simulink model "oldVers_1704_old"  (R2023a)
settings: Solver=ode1  StartTime=0.0  StopTime=0.5  FixedStep=0.000001  RelTol=1e-3
values from neighbouring files (symbols this model uses):
  Cm = 0.05    [matlab2.mat]
  Jm = 1    [matlab2.mat]
  k_eq = 1    [matlab2.mat]
  k_pos = 1    [matlab2.mat]
  Ki_Curr = 1666    [matlab2.mat]
  Kinv = 18    [matlab2.mat]
  Kp_Curr = 0.0229017    [matlab2.mat]
  Re = 0.357267    [matlab2.mat]
  T_eq = 0.00052    [matlab2.mat]
  T_eq2 = 0.0018    [matlab2.mat]
  Te = 0.0006    [matlab2.mat]
  Tinv = 0.00026    [matlab2.mat]
undefined symbols (not defined in the file or in its folder): Kc_Curr, Kc_Pos, Kc_Speed, Kis_Curr
libraries: simulink x3
settings Model: Creator=Ruslan  LastModifiedBy=sokur
settings SolverCC: AlgebraicLoopSolver=TrustRegion
settings ModelReferenceCC: EnableRefExpFcnMdlSchedulingChecks=on

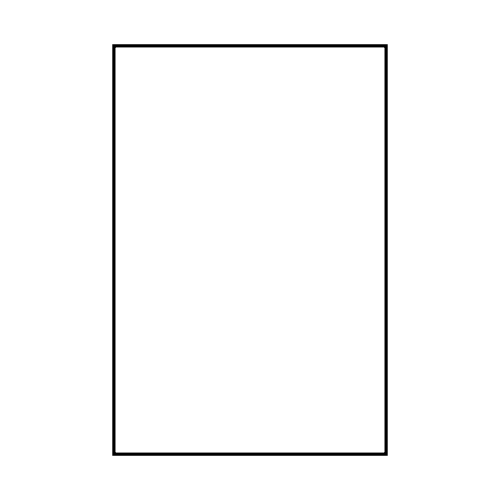
[thumbnail: Simulink's stored preview of the top-level diagram]
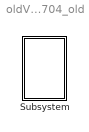
== system oldVers_1704_old ==
  Subsystem : Subsystem

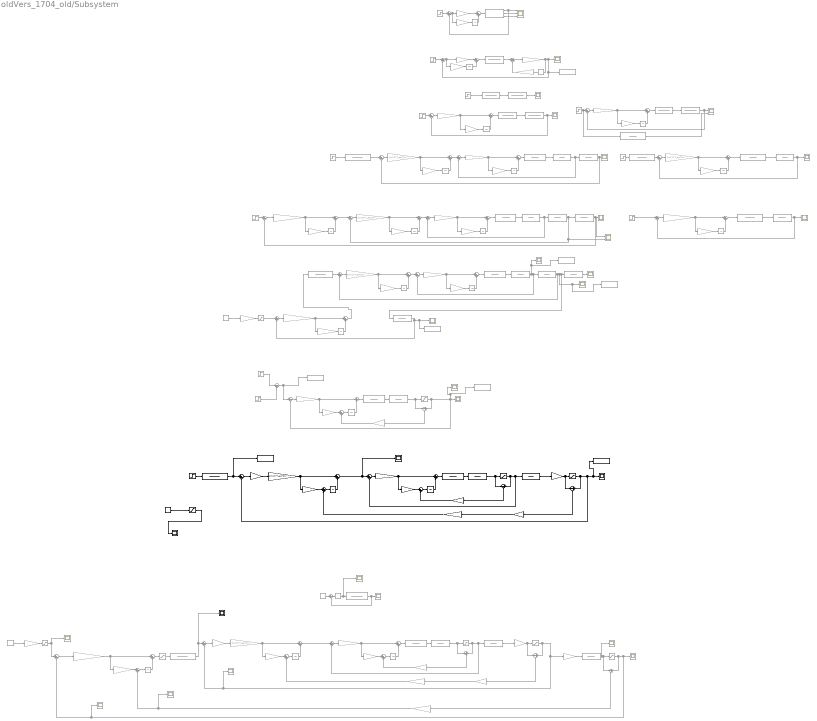
== system oldVers_1704_old/Subsystem ==
  note: Контур скорости с насыщениями рабочий
  note: Контур тока с ограничениями рабочий
  note: Контур положения рабочий
  note: Контур скорости
  note: Контур тока
  note: Контур тока
  note: Контур тока рабочий
  1 : TransferFcn  Commented=on  Numerator=[Cm]  Denominator=[Jm 0]
  1/Rяц : Gain  Commented=on  Gain=1/0.357267
  2 : TransferFcn  Commented=on  Numerator=[k_pos]  Denominator=[1 0]
  3 : TransferFcn  Commented=on  Numerator=[k_pos]  Denominator=[1 0]
  Constant : Constant  Commented=on  Value=20
  Derivative : Derivative  Commented=on
  Integrator{,1..14,19..20,22} (18 alike) : Integrator  Commented=on
  Integrator16 : Integrator
  Integrator18 : Integrator
  Kп : Gain  Commented=on  Gain=0.00067
  Kп1 : Gain  Commented=on  Gain=0.00067
  Kп{6,10..11,32} (4 alike) : Gain  Commented=on  Gain=(1)/(2*T_eq2*k_pos)
  Kп{3,8,12..13,25} (5 alike) : Gain  Commented=on  Gain=Kp_Curr
  Kп{4,7,9,14,27} (5 alike) : Gain  Commented=on  Gain=(Jm)/(2*T_eq*Cm)
  Kп2 : Gain  Commented=on  Gain=0.0229017
  Kп20 : Gain  Gain=Kp_Curr
  Kп21 : Gain  Gain=30/pi
  Kп22 : Gain  Gain=(Jm)/(2*T_eq*Cm)
  Kп23 : Gain  Gain=1/(30/pi)
  Kп24 : Gain  Gain=1/(30/pi)
  Kп26 : Gain  Commented=on  Gain=30/pi
  Kп28 : Gain  Commented=on  Gain=1/(30/pi)
  Kп29 : Gain  Commented=on  Gain=1/(30/pi)
  Kп33 : Gain  Commented=on  Gain=1/(30/pi)
  Kп5 : Gain  Commented=on  Gain=0.0229017
  L : Gain  Commented=on  Gain=0.001457602
  Ramp1 : simulink/Sources/Ramp  Commented=on  slope=120  start=0  InitialOutput=0
  Ramp2 : simulink/Sources/Ramp  Commented=on  slope=10000  start=0  InitialOutput=0
  Ramp3 : simulink/Sources/Ramp  slope=7500  start=0  InitialOutput=0
  Relay : Relay  Commented=on  OnOutputValue=20  OffOutputValue=-20
  Saturation : Saturate  Commented=on  UpperLimit=70  LowerLimit=-70
  Saturation1 : Saturate  Commented=on  UpperLimit=48  LowerLimit=-48
  Saturation10 : Saturate  UpperLimit=750  LowerLimit=-750
  Saturation2 : Saturate  Commented=on  UpperLimit=2000  LowerLimit=-2000
  Saturation4 : Saturate  UpperLimit=70  LowerLimit=-70
  Saturation5 : Saturate  UpperLimit=750  LowerLimit=-750
  Saturation6 : Saturate  Commented=on  UpperLimit=70  LowerLimit=-70
  Saturation7 : Saturate  Commented=on  UpperLimit=750  LowerLimit=-750
  Saturation8 : Saturate  Commented=on  UpperLimit=96  LowerLimit=-40
  Saturation9 : Saturate  Commented=on  UpperLimit=90  LowerLimit=-90
  Scope : Scope  Commented=on  NumInputPorts=3
  Scope{1..4,6..9,11..13,15..19,21,23..26} (21 alike) : Scope  Commented=on
  Scope10 : Scope  Commented=on  NumInputPorts=2
  Scope{14,20,22,27} (4 alike) : Scope
  Scope5 : Scope  Commented=on  NumInputPorts=2
  Step : Step  Commented=on  Time=0  After=-12  SampleTime=0
  Step{1..7,9} (8 alike) : Step  Commented=on  Time=0  SampleTime=0
  Step10 : Step  Commented=on  Time=0.0017  After=50  SampleTime=0
  Step11 : Step  Time=0  After=700  SampleTime=0
  Step8 : Step  Commented=on  Time=0  After=100  SampleTime=0
  Sum{,2,6,8..9,12,15..16,19..20,22,24,27..28,30,34,51,55,63} (19 alike) : Sum  Commented=on  Inputs=|+-
  Sum{1,3,5,7,10..11,13..14,17..18,21,23,25..26,29,31,50,52,54,56,62,65} (22 alike) : Sum  Commented=on  Inputs=|++
  Sum{32,53,57,64} (4 alike) : Sum  Commented=on  Inputs=-|+
  Sum33 : Sum  Commented=on  Inputs=|-+
  Sum4 : Sum  Commented=on  Inputs=-+-
  Sum{42,44,46,48} (4 alike) : Sum  Inputs=|++
  Sum43 : Sum  Inputs=|+-
  Sum45 : Sum  Inputs=-|+
  Sum47 : Sum  Inputs=|+-
  Sum49 : Sum  Inputs=-|+
  To Workspace : ToWorkspace  Commented=on  VariableName=simout  SaveFormat=Timeseries  SampleTime=-1
  To Workspace1 : ToWorkspace  Commented=on  VariableName=pos  SaveFormat=Timeseries  SampleTime=-1
  To Workspace2 : ToWorkspace  Commented=on  VariableName=posCurr  SaveFormat=Timeseries  SampleTime=-1
  To Workspace3 : ToWorkspace  Commented=on  VariableName=posSpd  SaveFormat=Timeseries  SampleTime=-1
  To Workspace4 : ToWorkspace  Commented=on  VariableName=CurrC  SaveFormat=Timeseries  SampleTime=-1
  To Workspace5 : ToWorkspace  Commented=on  VariableName=CurrCRef  SaveFormat=Timeseries  SampleTime=-1
  To Workspace6 : ToWorkspace  VariableName=SpdC  SaveFormat=Timeseries  SampleTime=-1
  To Workspace7 : ToWorkspace  VariableName=SpdCRef  SaveFormat=Timeseries  SampleTime=-1
  Transfer Fcn : TransferFcn  Commented=on  Denominator=[Kis_Curr 0]
  Аппроксимация ЗКС : TransferFcn  Commented=on  Denominator=[T_eq2 1]
  Аппроксимация ЗКТ : TransferFcn  Commented=on  Numerator=[k_eq]  Denominator=[T_eq 1]
  Аппроксимация ЗКТ1 : TransferFcn  Commented=on  Denominator=[T_eq 1]
  Аппроксимация ЗКТ3 : TransferFcn  Commented=on  Denominator=[4*T_eq 1]
  ДПТ : Subsystem  Commented=on
  Инвентор : TransferFcn  Commented=on  Numerator=[617.143]  Denominator=[0.00026 1]
  Инвентор1 : TransferFcn  Commented=on  Numerator=[18]  Denominator=[0.00026 1]
  Инвентор{3,5..6,8,10} (5 alike) : TransferFcn  Commented=on  Numerator=[Kinv]  Denominator=[Tinv 1]
  Инвентор2 : TransferFcn  Commented=on  Numerator=[18]  Denominator=[0.00026 1]
  Инвентор4 : TransferFcn  Commented=on  Numerator=[18]  Denominator=[0.00026 1]
  Инвентор9 : TransferFcn  Numerator=[Kinv]  Denominator=[Tinv 1]
  Ки : Gain  Commented=on  Gain=0.22167
  Ки1 : Gain  Commented=on  Gain=0.22167
  Ки{6,10..11,31} (4 alike) : Gain  Commented=on  Gain=1/(4*T_eq2)
  Ки12 : Gain  Commented=on  Gain=Kc_Curr
  Ки{3,8,13..14,26} (5 alike) : Gain  Commented=on  Gain=Ki_Curr
  Ки{4,7,9,15,28} (5 alike) : Gain  Commented=on  Gain=1/(4*T_eq)
  Ки16 : Gain  Commented=on  Gain=1/k_pos
  Ки2 : Gain  Commented=on  Gain=1666
  Ки21 : Gain  Gain=Kc_Curr
  Ки22 : Gain  Gain=Ki_Curr
  Ки23 : Gain  Gain=Kc_Speed
  Ки24 : Gain  Gain=1/(4*T_eq)
  Ки25 : Gain  Commented=on  Gain=Kc_Curr
  Ки27 : Gain  Commented=on  Gain=Kc_Speed
  Ки29 : Gain  Commented=on  Gain=1/k_pos
  Ки32 : Gain  Commented=on  Gain=Kc_Pos
  Ки5 : Gain  Commented=on  Gain=1666
  Оптимизирующее звено : TransferFcn  Commented=on  Denominator=[4*T_eq 1]
  Оптимизирующее звено1 : TransferFcn  Denominator=[4*T_eq 1]
  Оптимизирующее звено2 : TransferFcn  Commented=on  Denominator=[4*T_eq 1]
  Оптимизирующий фильтр : TransferFcn  Commented=on  Denominator=[4*T_eq 1]
  мех сост{,1..2,5} (4 alike) : TransferFcn  Commented=on  Numerator=[Cm]  Denominator=[Jm 0]
  мех сост4 : TransferFcn  Numerator=[Cm]  Denominator=[Jm 0]
  полож : TransferFcn  Commented=on  Numerator=[k_pos]  Denominator=[1 0]
  полож1 : TransferFcn  Commented=on  Numerator=[k_pos]  Denominator=[1 0]
  полож3 : TransferFcn  Commented=on  Numerator=[k_pos]  Denominator=[1 0]
  электромагнит сост : TransferFcn  Commented=on  Numerator=[1/0.357267]  Denominator=[0.0006 1]
  электромагнит сост1 : TransferFcn  Commented=on  Numerator=[1/0.357267]  Denominator=[0.0006 1]
  электромагнит сост{2,4..5,7,9} (5 alike) : TransferFcn  Commented=on  Numerator=[1/Re]  Denominator=[Te 1]
  электромагнит сост3 : TransferFcn  Commented=on  Numerator=[1/0.357267]  Denominator=[0.0006 1]
  электромагнит сост8 : TransferFcn  Numerator=[1/Re]  Denominator=[Te 1]
  wires:
  Sum/1 -> Kп/1, Ки/1
  Sum1/1 -> ДПТ/1(Uвх)
  Ки/1 -> Integrator/1
  Step/1 -> Sum/1
  Kп/1 -> Sum1/1
  ДПТ/1(I) -> Sum/2, Scope/1
  ДПТ/3(M) -> Scope/3
  Integrator/1 -> Sum1/2
  ДПТ/2(ω) -> Scope/2
  Integrator1/1 -> Sum3/2
  Sum2/1 -> Kп1/1, Ки1/1
  Kп1/1 -> Sum3/1
  Ки1/1 -> Integrator1/1
  Step1/1 -> Sum2/1
  Sum4/1 -> 1/Rяц/1
  L/1 -> Sum4/3
  Derivative/1 -> L/1
  1/Rяц/1 -> Derivative/1, To Workspace/1, Sum2/2, Scope2/1  "Iя"
  Sum3/1 -> Инвентор/1
  Инвентор/1 -> Sum4/2
  Step2/1 -> Инвентор1/1
  Инвентор1/1 -> электромагнит сост/1
  электромагнит сост/1 -> Scope1/1
  Инвентор2/1 -> электромагнит сост1/1
  электромагнит сост1/1 -> Scope3/1, Sum6/2
  Ки2/1 -> Integrator2/1
  Integrator2/1 -> Sum5/2
  Kп2/1 -> Sum5/1, Ки2/1
  Sum5/1 -> Инвентор2/1
  Step3/1 -> Sum6/1
  Sum6/1 -> Kп2/1
  Kп3/1 -> Sum7/1, Ки3/1
  Integrator3/1 -> Sum7/2
  Sum8/1 -> Kп3/1
  электромагнит сост2/1 -> мех сост/1, Sum8/2
  Инвентор3/1 -> электромагнит сост2/1
  Sum7/1 -> Инвентор3/1
  Ки3/1 -> Integrator3/1
  Kп4/1 -> Ки4/1, Sum10/1
  Integrator4/1 -> Sum10/2
  Ки4/1 -> Integrator4/1
  Sum9/1 -> Kп4/1
  Sum10/1 -> Sum8/1
  мех сост/1 -> Sum9/2, Scope4/1
  Kп5/1 -> Sum11/1, Ки5/1
  Integrator5/1 -> Sum11/2
  Sum12/1 -> Kп5/1
  Step5/1 -> Аппроксимация ЗКТ/1, Sum12/1
  электромагнит сост3/1 -> Scope5/1, Sum12/2
  Инвентор4/1 -> электромагнит сост3/1
  Sum11/1 -> Инвентор4/1
  Ки5/1 -> Integrator5/1
  Аппроксимация ЗКТ/1 -> Scope5/2
  Ки9/1 -> Integrator9/1
  Integrator9/1 -> Sum17/2
  Kп9/1 -> Ки9/1, Sum17/1
  Sum20/1 -> Kп9/1
  мех сост2/1 -> Scope10/2, Sum20/2, полож/1
  Integrator8/1 -> Sum18/2
  Sum19/1 -> Kп8/1
  Sum17/1 -> Sum19/1
  Kп8/1 -> Sum18/1, Ки8/1
  Инвентор6/1 -> электромагнит сост5/1
  Sum18/1 -> Инвентор6/1
  электромагнит сост5/1 -> мех сост2/1, Sum19/2
  Ки8/1 -> Integrator8/1
  Integrator10/1 -> Sum21/2
  Kп10/1 -> Ки10/1, Sum21/1
  Ки10/1 -> Integrator10/1
  полож/1 -> Sum22/2, Scope10/1, Scope7/1
  Sum22/1 -> Kп10/1
  Ки7/1 -> Integrator7/1
  Sum13/1 -> Аппроксимация ЗКТ1/1
  Kп7/1 -> Ки7/1, Sum13/1
  Sum16/1 -> Kп7/1
  Аппроксимация ЗКТ1/1 -> 1/1
  Integrator7/1 -> Sum13/2
  1/1 -> Scope6/1, Sum16/2
  Step6/1 -> Аппроксимация ЗКТ3/1
  Аппроксимация ЗКТ3/1 -> Sum16/1
  Step4/1 -> Оптимизирующий фильтр/1
  Оптимизирующий фильтр/1 -> Sum9/1
  2/1 -> Scope9/1, Sum15/2
  Sum14/1 -> Аппроксимация ЗКС/1
  Ки6/1 -> Integrator6/1
  Kп6/1 -> Ки6/1, Sum14/1
  Sum15/1 -> Kп6/1
  Integrator6/1 -> Sum14/2
  Step9/1 -> Sum15/1
  Аппроксимация ЗКС/1 -> 2/1
  Sum21/1 -> Sum20/1
  Step7/1 -> Sum22/1
  Kп11/1 -> Ки11/1, Sum23/1
  Sum24/1 -> Kп11/1
  Sum23/1 -> Оптимизирующее звено/1
  3/1 -> To Workspace1/1, Scope8/1, Sum24/2
  Integrator11/1 -> Sum23/2
  Ки11/1 -> Integrator11/1
  Sum28/1 -> Kп14/1
  Инвентор5/1 -> электромагнит сост4/1
  электромагнит сост4/1 -> Scope24/1, To Workspace2/1, мех сост1/1, Sum27/2
  Kп14/1 -> Ки15/1, Sum25/1
  Ки14/1 -> Integrator13/1
  Integrator13/1 -> Sum26/2
  Sum26/1 -> Инвентор5/1
  Sum27/1 -> Kп13/1
  Kп13/1 -> Sum26/1, Ки14/1
  Integrator14/1 -> Sum25/2
  Sum25/1 -> Sum27/1
  полож1/1 -> Scope12/1
  Ки15/1 -> Integrator14/1
  Ки16/1 -> Saturation1/1
  Ramp1/1 -> Ки16/1
  Оптимизирующее звено/1 -> Sum28/1
  Sum29/1 -> Инвентор8/1
  Integrator12/1 -> Sum29/2
  Инвентор8/1 -> электромагнит сост7/1
  Kп12/1 -> Ки13/1, Sum29/1
  электромагнит сост7/1 -> Sum32/1, Saturation/1
  Sum30/1 -> Kп12/1
  Sum31/1 -> Integrator12/1
  Ки13/1 -> Sum31/1
  Sum32/1 -> Ки12/1
  Step8/1 -> Sum33/2
  Step10/1 -> Sum33/1
  Ки12/1 -> Sum31/2
  Sum65/1 -> Integrator22/1
  Saturation9/1 -> Sum64/2, Scope15/1, Scope18/1, Sum63/2
  полож3/1 -> Scope16/1, Sum64/1, Saturation9/1
  Ки31/1 -> Sum65/1
  Ки32/1 -> Scope17/1, Sum65/2
  Kп33/1 -> полож3/1
  Integrator22/1 -> Sum62/2
  Kп32/1 -> Ки31/1, Sum62/1
  Sum64/1 -> Ки32/1
  Sum63/1 -> Kп32/1
  Saturation5/1 -> Sum49/2, To Workspace6/1, Scope14/1, Sum47/2
  Saturation4/1 -> Sum45/2, мех сост4/1, Sum43/2
  мех сост4/1 -> Kп21/1
  Ки21/1 -> Sum44/2
  Sum44/1 -> Integrator16/1
  Sum47/1 -> Kп23/1
  Ки24/1 -> Sum48/1
  Ки23/1 -> Sum48/2
  Kп24/1 -> Ки23/1
  Step11/1 -> Оптимизирующее звено1/1
  Sum46/1 -> Scope27/1, Sum43/1
  Integrator18/1 -> Sum46/2
  Integrator16/1 -> Sum42/2
  Kп22/1 -> Ки24/1, Sum46/1
  Sum49/1 -> Kп24/1
  Sum45/1 -> Ки21/1
  Инвентор9/1 -> электромагнит сост8/1
  электромагнит сост8/1 -> Sum45/1, Saturation4/1
  Kп20/1 -> Ки22/1, Sum42/1
  Sum43/1 -> Kп20/1
  Ки22/1 -> Sum44/1
  Sum48/1 -> Integrator18/1
  Kп23/1 -> Kп22/1
  Sum42/1 -> Инвентор9/1
  Kп21/1 -> Sum49/1, Saturation5/1
  Kп26/1 -> Sum57/1, Saturation7/1
  Sum53/1 -> Ки25/1
  Ки26/1 -> Sum52/1
  Sum57/1 -> Kп29/1
  электромагнит сост9/1 -> Sum53/1, Saturation6/1
  Sum50/1 -> Инвентор10/1
  Инвентор10/1 -> электромагнит сост9/1
  Integrator19/1 -> Sum50/2
  Sum54/1 -> Sum51/1
  Integrator20/1 -> Sum54/2
  Sum52/1 -> Integrator19/1
  Ки27/1 -> Sum56/2
  Ки28/1 -> Sum56/1
  Kп29/1 -> Ки27/1
  Kп27/1 -> Ки28/1, Sum54/1
  Kп25/1 -> Ки26/1, Sum50/1
  Saturation2/1 -> Оптимизирующее звено2/1
  Sum56/1 -> Integrator20/1
  Ки25/1 -> Sum52/2
  Sum51/1 -> Kп25/1
  Sum55/1 -> Kп28/1
  мех сост5/1 -> Kп26/1
  Kп28/1 -> Kп27/1
  Saturation6/1 -> Sum53/2, мех сост5/1, Sum51/2
  Saturation7/1 -> Sum57/2, Kп33/1, Scope21/1, Sum55/2
  Ки29/1 -> Saturation8/1
  Ramp2/1 -> Ки29/1
  Saturation8/1 -> Sum63/1, Scope19/1
  Ramp3/1 -> Saturation10/1
  Saturation10/1 -> Scope22/1
  Sum62/1 -> Saturation2/1
  Relay/1 -> Scope23/1, Transfer Fcn/1
  Transfer Fcn/1 -> Sum34/2, Scope13/1
  Constant/1 -> Sum34/1
  Sum34/1 -> Relay/1
  Оптимизирующее звено2/1 -> Scope20/1, Sum55/1
  Saturation1/1 -> Sum24/1
  мех сост1/1 -> Sum28/2, To Workspace3/1, Scope25/1, 3/1, полож1/1
  Saturation/1 -> Sum32/2, To Workspace4/1, Scope26/1, Scope11/1, Sum30/2
  Sum33/1 -> To Workspace5/1, Sum30/1
  Оптимизирующее звено1/1 -> To Workspace7/1, Sum47/1

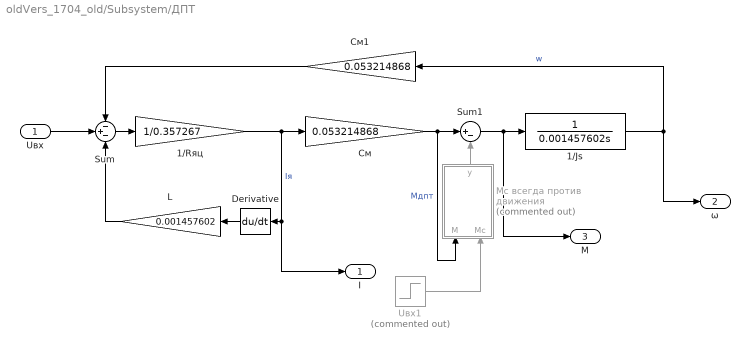
== system oldVers_1704_old/Subsystem/ДПТ ==
  Uвх : Inport
  1/Js : TransferFcn  Denominator=[0.001457602 0]
  1/Rяц : Gain  Gain=1/0.357267
  Cм : Gain  Gain=0.053214868
  Cм1 : Gain  Gain=0.053214868
  Derivative : Derivative
  L : Gain  Gain=0.001457602
  Sum : Sum  Inputs=-+-
  Sum1 : Sum  Inputs=|+-
  Uвх1 : Step  Commented=on  After=0.06  SampleTime=0
  Мс всегда против движения : MATLAB Function  Commented=on  TreatAsAtomicUnit=on
  I : Outport
  ω : Outport  Port=2
  M : Outport  Port=3
  wires:
  1/Rяц/1 -> I/1, Derivative/1, Cм/1  "Iя"
  Uвх/1 -> Sum/2
  L/1 -> Sum/3
  1/Js/1 -> Cм1/1, ω/1  "w"
  Cм1/1 -> Sum/1
  Derivative/1 -> L/1
  Sum1/1 -> M/1, 1/Js/1
  Uвх1/1 -> Мс всегда против движения/2(Mc)
  Sum/1 -> 1/Rяц/1
  Cм/1 -> Мс всегда против движения/1(M), Sum1/1  "Мдпт"
  Мс всегда против движения/1(y) -> Sum1/2

== matlab function oldVers_1704_old/Subsystem/ДПТ/Мс всегда против движения ==
  data: M input; Mc input; y output
function y = fcn(M, Mc)
if (M>0)
    y = Mc;
else
    y = -Mc;
end
